simulink model "Loads"  (R2025b)
settings: Solver=VariableStepAuto  StartTime=0.0  StopTime=10.0  RelTol=1e-3
model workspace (MAT data in the model file):
  actuator_load_matrix = [745.046606557 524.370349362 302.714903905 163.595100453 62.8616081905 7.8273147351 0 38.8629907274 123.372985084 247.793030257 405.167536851 587.013620169 ... (280 elements, 14x20)]
  aileron_deflections_deg = [-30 -25 -20 -15 -10 -5 0 5 10 15 20 25 30 35]
  airspeeds_mps = [70 78.9473684211 87.8947368421 96.8421052632 105.789473684 114.736842105 123.684210526 132.631578947 141.578947368 150.526315789 159.473684211 168.421052632 177.368421053 186.315789474 195.263157895 204.210526316 213.157894737 222.105263158 231.052631579 240]
settings Model: Creator=ikita  LastModifiedBy=mikol

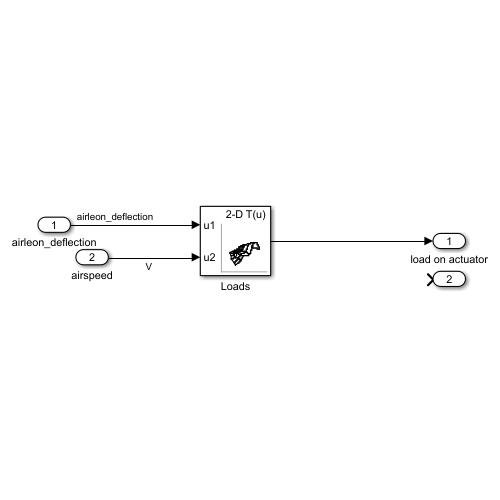
[thumbnail: Simulink's stored preview of the top-level diagram]
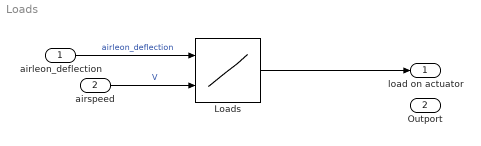
== system Loads ==
  airleon_deflection : Inport
  airspeed : Inport  Port=2
  Loads : Lookup_n-D  BreakpointsForDimension1=aileron_deflections_deg  BreakpointsForDimension2=airspeeds_mps  Table=actuator_load_matrix  InterpMethod=Cubic spline  ExtrapMethod=Cubic spline  DiagnosticForOutOfRangeInput=Warning  InternalRulePriority=Speed  RndMeth=Simplest
      settings: InputPortMap=u0,u1
  load on actuator : Outport
  Outport : Outport  Port=2
  wires:
  airleon_deflection/1 -> Loads/1  "airleon_deflection"
  airspeed/1 -> Loads/2  "V"
  Loads/1 -> load on actuator/1
